simulink model "sequence_generator"  (R2025b)
settings: Solver=VariableStepAuto  StartTime=0.0  StopTime=10.0  RelTol=1e-3
libraries: simulink_extras x4
settings Model: Creator=Johan  LastModifiedBy=Johan

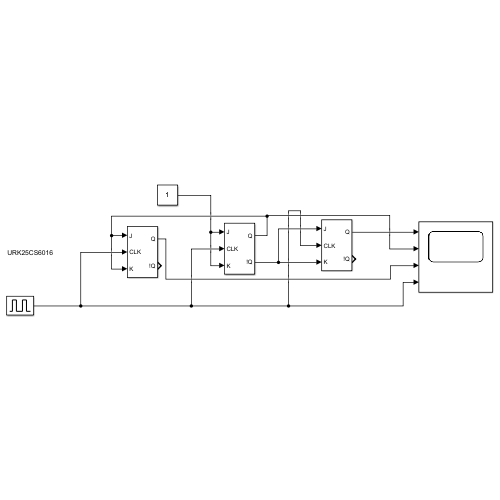
[thumbnail: Simulink's stored preview of the top-level diagram]
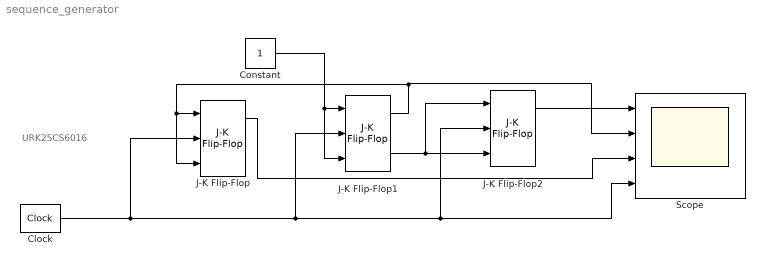
== system sequence_generator ==
  note: URK25CS6016
  Clock : simulink_extras/Flip Flops/Clock  period=2
  Constant : Constant  OutDataTypeStr=boolean
  J-K Flip-Flop : simulink_extras/Flip Flops/J-K Flip-Flop  initial_condition=0
  J-K Flip-Flop1 : simulink_extras/Flip Flops/J-K Flip-Flop  initial_condition=0
  J-K Flip-Flop2 : simulink_extras/Flip Flops/J-K Flip-Flop  initial_condition=0
  Scope : Scope  NumInputPorts=4
      settings: ActiveDisplayYMinimum=-0.12499999999999997  ActiveDisplayYMaximum=1.125
  wires:
  Clock/1 -> Scope/4, J-K Flip-Flop2/2, J-K Flip-Flop1/2, J-K Flip-Flop/2
  J-K Flip-Flop1/2 -> J-K Flip-Flop2/1, J-K Flip-Flop2/3
  J-K Flip-Flop/1 -> Scope/3
  J-K Flip-Flop1/1 -> J-K Flip-Flop/3, J-K Flip-Flop/1, Scope/2
  J-K Flip-Flop2/1 -> Scope/1
  Constant/1 -> J-K Flip-Flop1/3, J-K Flip-Flop1/1
